simulink model "com_recieve_video"  (R2016b)
settings: Solver=VariableStepAuto  StartTime=0.0  StopTime=10.0  RelTol=1e-3
libraries: etargetslib x5, dspnetwork x5
settings Model: Creator=zeabus  LastModifiedBy=zeabus

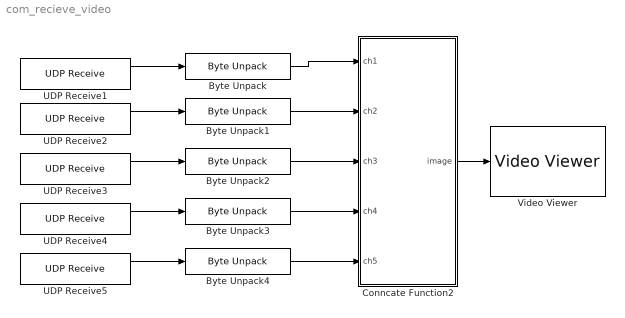
== system com_recieve_video ==
  Byte Unpack{,1..4} (5 alike) : etargetslib/Byte Unpack  dimensions={[15360]}  datatypes={'uint8'}  byteAlign=1
  Conncate Function2 : MATLAB Function  TreatAsAtomicUnit=on
  UDP Receive1 : dspnetwork/UDP Receive  localURL='0.0.0.0'  localPort=30000  remoteURL='10.2.12.154'  remotePort=-1  recvBufferSize=61500  dims=15360  signalDatatype=uint8  isVarSize=off  showBlockingTime=on  blockingTime=0.01  sampletime=0.01  blockPlatform=HOST
  UDP Receive2 : dspnetwork/UDP Receive  localURL='0.0.0.0'  localPort=30001  remoteURL='10.2.12.154'  remotePort=-1  recvBufferSize=61500  dims=15360  signalDatatype=uint8  isVarSize=off  showBlockingTime=on  blockingTime=0.01  sampletime=0.01  blockPlatform=HOST
  UDP Receive3 : dspnetwork/UDP Receive  localURL='0.0.0.0'  localPort=30002  remoteURL='10.2.12.154'  remotePort=-1  recvBufferSize=61500  dims=15360  signalDatatype=uint8  isVarSize=off  showBlockingTime=on  blockingTime=0.01  sampletime=0.01  blockPlatform=HOST
  UDP Receive4 : dspnetwork/UDP Receive  localURL='0.0.0.0'  localPort=30003  remoteURL='10.2.12.154'  remotePort=-1  recvBufferSize=61500  dims=15360  signalDatatype=uint8  isVarSize=off  showBlockingTime=on  blockingTime=0.01  sampletime=0.01  blockPlatform=HOST
  UDP Receive5 : dspnetwork/UDP Receive  localURL='0.0.0.0'  localPort=30004  remoteURL='10.2.12.154'  remotePort=-1  recvBufferSize=61500  dims=15360  signalDatatype=uint8  isVarSize=off  showBlockingTime=on  blockingTime=0.01  sampletime=0.01  blockPlatform=HOST
  Video Viewer : VideoViewer  FigPos=[765 846 905 545]
  wires:
  UDP Receive1/1 -> Byte Unpack/1
  UDP Receive2/1 -> Byte Unpack1/1
  UDP Receive3/1 -> Byte Unpack2/1
  UDP Receive4/1 -> Byte Unpack3/1
  UDP Receive5/1 -> Byte Unpack4/1
  Byte Unpack3/1 -> Conncate Function2/4(ch4)
  Byte Unpack4/1 -> Conncate Function2/5(ch5)
  Byte Unpack2/1 -> Conncate Function2/3(ch3)
  Byte Unpack1/1 -> Conncate Function2/2(ch2)
  Byte Unpack/1 -> Conncate Function2/1(ch1)
  Conncate Function2/1(image) -> Video Viewer/1

== matlab function com_recieve_video/Conncate Function2 ==
  data: ch1 input; ch2 input; ch3 input; ch4 input; ch5 input uint8; image output
function image  = concatenation(ch1,ch2,ch3,ch4,ch5)
maxcol = 48;
height = 320;
width = 240;
ch1 = reshape(ch1,height,maxcol);
ch2 = reshape(ch2,height,maxcol);
ch3 = reshape(ch3,height,maxcol);
ch4 = reshape(ch4,height,maxcol);
ch5 = reshape(ch5,height,maxcol);
image = [ch1,ch2,ch3,ch4,ch5];
image = reshape(image,height,width);
